simulink model "Copy_of_project_RFT_DataGen2020a"  (R2021b)
settings: Solver=ode4  StartTime=0.0  StopTime=7  FixedStep=0.0001  MaxStep=1e-4  RelTol=1e-5
settings Model: Creator=Mohamad Chehadeh  LastModifiedBy=Admin
settings SolverCC: AlgebraicLoopSolver=TrustRegion
settings DebuggingCC: SFMachineParentedDataDiag=warning

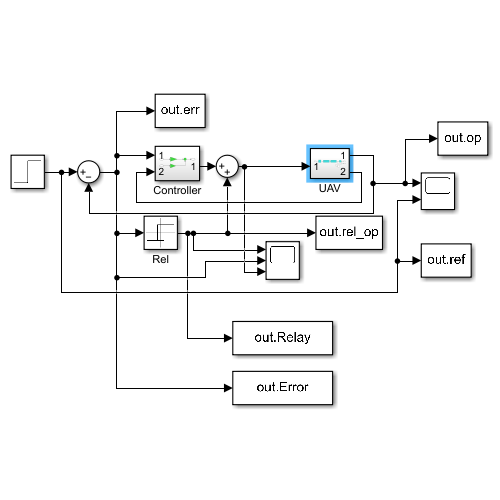
[thumbnail: Simulink's stored preview of the top-level diagram]
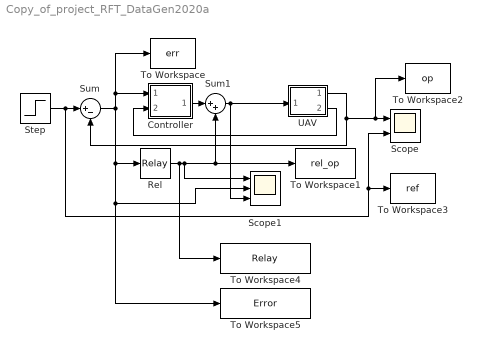
== system Copy_of_project_RFT_DataGen2020a ==
  Controller : Subsystem
  Rel : Relay  OffSwitchValue=-eps  OffOutputValue=-1
  Scope : Scope  NumInputPorts=2
  Scope1 : Scope  NumInputPorts=3
  Step : Step  SampleTime=0
  Sum : Sum  Inputs=|+-
  Sum1 : Sum  Inputs=|++
  To Workspace : ToWorkspace  VariableName=err  SaveFormat=Timeseries  SampleTime=-1
  To Workspace1 : ToWorkspace  VariableName=rel_op  SaveFormat=Timeseries  SampleTime=-1
  To Workspace2 : ToWorkspace  VariableName=op  SaveFormat=Timeseries  SampleTime=-1
  To Workspace3 : ToWorkspace  VariableName=ref  SaveFormat=Timeseries  SampleTime=-1
  To Workspace4 : ToWorkspace  VariableName=Relay  SampleTime=-1
  To Workspace5 : ToWorkspace  VariableName=Error  SampleTime=-1
  UAV : Subsystem
  wires:
  Sum/1 -> To Workspace5/1, Scope1/2, Rel/1, To Workspace/1, Controller/1(In1)
  UAV/1(Out1) -> Sum/2, To Workspace2/1, Scope/1
  UAV/2(Out2) -> Controller/2(In2)
  Controller/1(Out1) -> Sum1/1
  Rel/1 -> To Workspace4/1, Scope1/1, To Workspace1/1, Sum1/2
  Step/1 -> Scope/2, To Workspace3/1, Sum/1
  Sum1/1 -> UAV/1(In1), Scope1/3

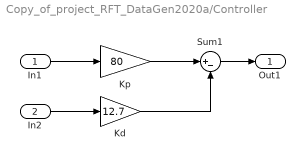
== system Copy_of_project_RFT_DataGen2020a/Controller ==
  In1 : Inport
  In2 : Inport  Port=2
  Kd : Gain  Gain=12.7
  Kp : Gain  Gain=80
  Sum1 : Sum  Inputs=|+-
  Out1 : Outport
  wires:
  In1/1 -> Kp/1
  Kp/1 -> Sum1/1
  In2/1 -> Kd/1
  Sum1/1 -> Out1/1
  Kd/1 -> Sum1/2

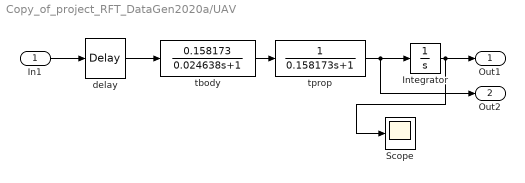
== system Copy_of_project_RFT_DataGen2020a/UAV ==
  In1 : Inport
  Integrator : Integrator
  Scope : Scope
  delay : TransportDelay  DelayTime=0.0607739
  tbody : TransferFcn  Numerator=0.158173  Denominator=[0.024638 1]
  tprop : TransferFcn  Denominator=[0.158173 1]
  Out1 : Outport
  Out2 : Outport  Port=2
  wires:
  tbody/1 -> tprop/1
  In1/1 -> delay/1
  tprop/1 -> Out2/1, Integrator/1
  delay/1 -> tbody/1
  Integrator/1 -> Scope/1, Out1/1
